simulink model "poop"  (R2019a)
settings: Solver=ode15s  StartTime=0.0  StopTime=0.2  RelTol=1e-3
values from neighbouring files (symbols this model uses):
  b = 3.5077E-6    (= 3.5077e-06)    [Controls_Project.m]
  J = 3.2284E-6    (= 3.2284e-06)    [Controls_Project.m]
  K = 0.0274    [Controls_Project.m]
  R = 4    [Controls_Project.m]
settings Model: Creator=rperez62  LastModifiedBy=rperez62

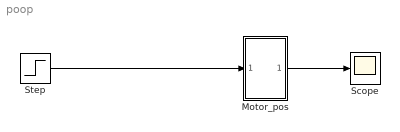
== system poop ==
  Motor_pos : Subsystem
  Scope : Scope
  Step : Step  Time=0  SampleTime=0
  wires:
  Step/1 -> Motor_pos/1(In1)
  Motor_pos/1(theta) -> Scope/1

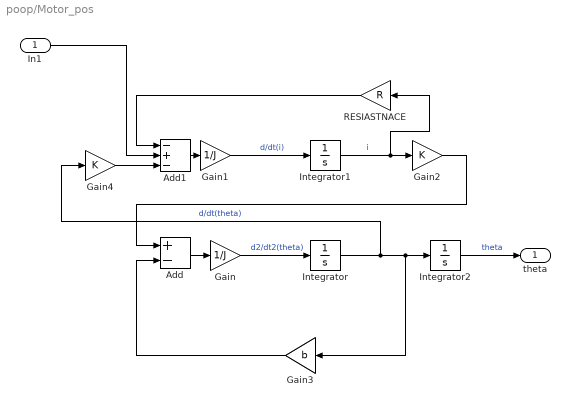
== system poop/Motor_pos ==
  In1 : Inport
  Add : Sum  Inputs=+-
  Add1 : Sum  Inputs=-+-
  Gain : Gain  Gain=1/J
  Gain1 : Gain  Gain=1/J
  Gain2 : Gain  Gain=K
  Gain3 : Gain  Gain=b
  Gain4 : Gain  Gain=K
  Integrator : Integrator
  Integrator1 : Integrator
  Integrator2 : Integrator
  RESIASTNACE : Gain  Gain=R
  theta : Outport
  wires:
  Add/1 -> Gain/1
  Gain3/1 -> Add/2
  RESIASTNACE/1 -> Add1/1
  Gain1/1 -> Integrator1/1  "d/dt(i)"
  Integrator1/1 -> RESIASTNACE/1, Gain2/1  "i"
  Integrator/1 -> Gain4/1, Gain3/1, Integrator2/1  "d/dt(theta)"
  Gain/1 -> Integrator/1  "d2/dt2(theta)"
  Gain2/1 -> Add/1
  Gain4/1 -> Add1/3
  Add1/1 -> Gain1/1
  Integrator2/1 -> theta/1  "theta"
  In1/1 -> Add1/2
